simulink model "IEEE14_case"  (R2024b)
settings: Solver=FixedStepAuto  StartTime=0  StopTime=2  FixedStep=1e-7  RelTol=1e-3
values from neighbouring files (symbols this model uses):
  GFL_15_Bva = 0.009    [IEEE14_parameters.m]
  GFL_15_C_bus_pu = 7.179419    [IEEE14_parameters.m]
  GFL_15_f0 = 60    [IEEE14_parameters.m]
  GFL_15_I_id = 691.26967    [IEEE14_parameters.m]
  GFL_15_I_iq = 691.26967    [IEEE14_parameters.m]
  GFL_15_I_od = 45.2207    [IEEE14_parameters.m]
  GFL_15_I_oq = 45.2207    [IEEE14_parameters.m]
  GFL_15_I_pll = 0.78    [IEEE14_parameters.m]
  GFL_15_Kdi = 0.09    [IEEE14_parameters.m]
  GFL_15_Kdo = 0.9    [IEEE14_parameters.m]
  GFL_15_Kqi = 0.09    [IEEE14_parameters.m]
  GFL_15_Kqo = 0.9    [IEEE14_parameters.m]
  GFL_15_Lg_pu = 0.631447    [IEEE14_parameters.m]
  GFL_15_mode = 1    [IEEE14_parameters.m]
  GFL_15_P_id = 3.7166    [IEEE14_parameters.m]
  GFL_15_P_iq = 3.7166    [IEEE14_parameters.m]
  GFL_15_P_od = 0.4798    [IEEE14_parameters.m]
  GFL_15_P_oq = 0.4798    [IEEE14_parameters.m]
  GFL_15_P_pll = 290.42    [IEEE14_parameters.m]
  GFL_15_Qe_ref = 0.2    [IEEE14_parameters.m]
  GFL_15_Rg_pu = 0.024016    [IEEE14_parameters.m]
  GFL_15_Sbase = 1.000000e+4    (= 10000)    [IEEE14_parameters.m]
  GFL_15_Tdi = 0.01    [IEEE14_parameters.m]
  GFL_15_Tdo = 0.2    [IEEE14_parameters.m]
  GFL_15_Tqi = 0.01    [IEEE14_parameters.m]
  GFL_15_Tqo = 0.2    [IEEE14_parameters.m]
  GFL_15_Vbase = 380    [IEEE14_parameters.m]
  GFL_15_Vdc_ref = 1.011475    [IEEE14_parameters.m]
  GFL_15_Vdcbase = 700    [IEEE14_parameters.m]
  GFL_15_vq_ref = 0    [IEEE14_parameters.m]
  GFL_16_Bva = 0.002    [IEEE14_parameters.m]
  GFL_16_C_bus_pu = 7.179419    [IEEE14_parameters.m]
  GFL_16_f0 = 60    [IEEE14_parameters.m]
  GFL_16_I_id = 691.26967    [IEEE14_parameters.m]
  GFL_16_I_iq = 691.26967    [IEEE14_parameters.m]
  GFL_16_I_od = 45.2207    [IEEE14_parameters.m]
  GFL_16_I_oq = 45.2207    [IEEE14_parameters.m]
  GFL_16_I_pll = 0.78    [IEEE14_parameters.m]
  GFL_16_Kdi = 0.05    [IEEE14_parameters.m]
  GFL_16_Kdo = 0.5    [IEEE14_parameters.m]
  GFL_16_Kqi = 0.05    [IEEE14_parameters.m]
  GFL_16_Kqo = 0.5    [IEEE14_parameters.m]
  GFL_16_Lg_pu = 0.631447    [IEEE14_parameters.m]
  GFL_16_mode = 1    [IEEE14_parameters.m]
  GFL_16_P_id = 3.7166    [IEEE14_parameters.m]
  GFL_16_P_iq = 3.7166    [IEEE14_parameters.m]
  GFL_16_P_od = 0.4798    [IEEE14_parameters.m]
  GFL_16_P_oq = 0.4798    [IEEE14_parameters.m]
  GFL_16_P_pll = 290.42    [IEEE14_parameters.m]
  GFL_16_Qe_ref = 0.2    [IEEE14_parameters.m]
  GFL_16_Rg_pu = 0.024016    [IEEE14_parameters.m]
  GFL_16_Sbase = 1.000000e+4    (= 10000)    [IEEE14_parameters.m]
  GFL_16_Tdi = 0.01    [IEEE14_parameters.m]
  GFL_16_Tdo = 0.2    [IEEE14_parameters.m]
  GFL_16_Tqi = 0.01    [IEEE14_parameters.m]
  GFL_16_Tqo = 0.2    [IEEE14_parameters.m]
  GFL_16_Vbase = 380    [IEEE14_parameters.m]
  GFL_16_Vdc_ref = 1.01144    [IEEE14_parameters.m]
  GFL_16_Vdcbase = 700    [IEEE14_parameters.m]
  GFL_16_vq_ref = 0    [IEEE14_parameters.m]
  GFL_17_Bva = 0.002    [IEEE14_parameters.m]
  GFL_17_C_bus_pu = 7.179419    [IEEE14_parameters.m]
  GFL_17_f0 = 60    [IEEE14_parameters.m]
  GFL_17_I_id = 691.26967    [IEEE14_parameters.m]
  GFL_17_I_iq = 691.26967    [IEEE14_parameters.m]
  GFL_17_I_od = 45.2207    [IEEE14_parameters.m]
  GFL_17_I_oq = 45.2207    [IEEE14_parameters.m]
  GFL_17_I_pll = 0.78    [IEEE14_parameters.m]
  GFL_17_Kdi = 0.05    [IEEE14_parameters.m]
  GFL_17_Kdo = 0.5    [IEEE14_parameters.m]
  GFL_17_Kqi = 0.05    [IEEE14_parameters.m]
  GFL_17_Kqo = 0.5    [IEEE14_parameters.m]
  GFL_17_Lg_pu = 0.631447    [IEEE14_parameters.m]
  GFL_17_mode = 1    [IEEE14_parameters.m]
  GFL_17_P_id = 3.7166    [IEEE14_parameters.m]
  GFL_17_P_iq = 3.7166    [IEEE14_parameters.m]
  GFL_17_P_od = 0.4798    [IEEE14_parameters.m]
  GFL_17_P_oq = 0.4798    [IEEE14_parameters.m]
  GFL_17_P_pll = 290.42    [IEEE14_parameters.m]
  GFL_17_Qe_ref = 0.2    [IEEE14_parameters.m]
  GFL_17_Rg_pu = 0.024016    [IEEE14_parameters.m]
  GFL_17_Sbase = 1.000000e+4    (= 10000)    [IEEE14_parameters.m]
  GFL_17_Tdi = 0.01    [IEEE14_parameters.m]
  GFL_17_Tdo = 0.2    [IEEE14_parameters.m]
  GFL_17_Tqi = 0.01    [IEEE14_parameters.m]
  GFL_17_Tqo = 0.2    [IEEE14_parameters.m]
  GFL_17_Vbase = 380    [IEEE14_parameters.m]
  GFL_17_Vdc_ref = 1.011632    [IEEE14_parameters.m]
  GFL_17_Vdcbase = 700    [IEEE14_parameters.m]
  GFL_17_vq_ref = 0    [IEEE14_parameters.m]
  GFL_18_Bva = 0.002    [IEEE14_parameters.m]
  GFL_18_C_bus_pu = 7.179419    [IEEE14_parameters.m]
  GFL_18_f0 = 60    [IEEE14_parameters.m]
  GFL_18_I_id = 691.26967    [IEEE14_parameters.m]
  GFL_18_I_iq = 691.26967    [IEEE14_parameters.m]
  GFL_18_I_od = 45.2207    [IEEE14_parameters.m]
  GFL_18_I_oq = 45.2207    [IEEE14_parameters.m]
  GFL_18_I_pll = 0.78    [IEEE14_parameters.m]
  GFL_18_Kdi = 0.05    [IEEE14_parameters.m]
  GFL_18_Kdo = 0.5    [IEEE14_parameters.m]
  GFL_18_Kqi = 0.05    [IEEE14_parameters.m]
  GFL_18_Kqo = 0.5    [IEEE14_parameters.m]
  GFL_18_Lg_pu = 0.631447    [IEEE14_parameters.m]
  GFL_18_mode = 1    [IEEE14_parameters.m]
  GFL_18_P_id = 3.7166    [IEEE14_parameters.m]
  GFL_18_P_iq = 3.7166    [IEEE14_parameters.m]
  GFL_18_P_od = 0.4798    [IEEE14_parameters.m]
  GFL_18_P_oq = 0.4798    [IEEE14_parameters.m]
  GFL_18_P_pll = 290.42    [IEEE14_parameters.m]
  GFL_18_Qe_ref = 0.2    [IEEE14_parameters.m]
  GFL_18_Rg_pu = 0.024016    [IEEE14_parameters.m]
  GFL_18_Sbase = 1.000000e+4    (= 10000)    [IEEE14_parameters.m]
  GFL_18_Tdi = 0.01    [IEEE14_parameters.m]
  GFL_18_Tdo = 0.2    [IEEE14_parameters.m]
  GFL_18_Tqi = 0.01    [IEEE14_parameters.m]
  GFL_18_Tqo = 0.2    [IEEE14_parameters.m]
  GFL_18_Vbase = 380    [IEEE14_parameters.m]
  GFL_18_Vdc_ref = 1.011572    [IEEE14_parameters.m]
  GFL_18_Vdcbase = 700    [IEEE14_parameters.m]
  GFL_18_vq_ref = 0    [IEEE14_parameters.m]
  ... (+180 more)
(part 6 of 25)

== system IEEE14_case/AC_1/d_id_line_7_9_block ==
  note: d_id_line_7_9 in case14gfl
      | $376.991118430775\,\mathrm{iq}_{\mathrm{line},7,9}+3426.88045114785\,\mathrm{vd}_{\mathrm{bus},7}-3426.88045114785\,\mathrm{vd}_{\mathrm{bus},9}$
      | Automatically generated on 2025-10-09 21:39:39 .
  State_iq_line_7_9_66432 : Inport
  State_vd_bus_7_8bd9d : Inport  Port=2
  State_vd_bus_9_0bd7a : Inport  Port=3
  Add_05699 : Sum
  Constant_3426.88045114785_50b4f : Constant  Value=3426.88045114785
  Constant_3426.88045114785_9598e : Constant  Value=3426.88045114785
  Constant_376.991118430775_0858e : Constant  Value=376.991118430775
  Product_57b21 : Product
  Product_92e7d : Product
  Product_acf4f : Product
  Subtract_c4abe : Sum  Inputs=+-
  Blockout_d_id_line_7_9_bf772 : Outport
  wires:
  State_iq_line_7_9_66432/1 -> Product_57b21/2
  Constant_376.991118430775_0858e/1 -> Product_57b21/1
  Constant_3426.88045114785_50b4f/1 -> Product_92e7d/1
  Product_92e7d/1 -> Add_05699/2
  State_vd_bus_7_8bd9d/1 -> Product_92e7d/2
  Product_57b21/1 -> Add_05699/1
  Product_acf4f/1 -> Subtract_c4abe/2
  Constant_3426.88045114785_9598e/1 -> Product_acf4f/1
  State_vd_bus_9_0bd7a/1 -> Product_acf4f/2
  Add_05699/1 -> Subtract_c4abe/1
  Subtract_c4abe/1 -> Blockout_d_id_line_7_9_bf772/1

== system IEEE14_case/AC_1/d_id_line_9_10_block ==
  note: d_id_line_9_10 in case14gfl
      | $376.991118430775\,\mathrm{iq}_{\mathrm{line},9,10}-141.918194997431\,\mathrm{id}_{\mathrm{line},9,10}+4461.43335421036\,\mathrm{vd}_{\mathrm{bus},9}-4461.43335421036\,\mathrm{vd}_{\mathrm{bus},10}$
      | Automatically generated on 2025-10-09 21:39:41 .
  State_id_line_9_10_959cd : Inport
  State_iq_line_9_10_22e13 : Inport  Port=2
  State_vd_bus_10_33748 : Inport  Port=3
  State_vd_bus_9_919cb : Inport  Port=4
  Add_7717b : Sum
  Add_e4eab : Sum
  Constant_-141.918194997431_d6c81 : Constant  Value=-141.918194997431
  Constant_376.991118430775_9f4c1 : Constant  Value=376.991118430775
  Constant_4461.43335421036_3f7bf : Constant  Value=4461.43335421036
  Constant_4461.43335421036_5c0f1 : Constant  Value=4461.43335421036
  Product_24143 : Product
  Product_2f834 : Product
  Product_723bb : Product
  Product_a30df : Product
  Subtract_8e61d : Sum  Inputs=+-
  Blockout_d_id_line_9_10_ec156 : Outport
  wires:
  Constant_-141.918194997431_d6c81/1 -> Product_a30df/1
  Product_a30df/1 -> Add_7717b/1
  State_id_line_9_10_959cd/1 -> Product_a30df/2
  Constant_376.991118430775_9f4c1/1 -> Product_24143/1
  Product_24143/1 -> Add_7717b/2
  Product_723bb/1 -> Subtract_8e61d/2
  Constant_4461.43335421036_3f7bf/1 -> Product_723bb/1
  State_iq_line_9_10_22e13/1 -> Product_24143/2
  State_vd_bus_10_33748/1 -> Product_723bb/2
  Add_7717b/1 -> Subtract_8e61d/1
  Constant_4461.43335421036_5c0f1/1 -> Product_2f834/1
  State_vd_bus_9_919cb/1 -> Product_2f834/2
  Subtract_8e61d/1 -> Add_e4eab/1
  Product_2f834/1 -> Add_e4eab/2
  Add_e4eab/1 -> Blockout_d_id_line_9_10_ec156/1

== system IEEE14_case/AC_1/d_id_line_9_14_block ==
  note: d_id_line_9_14 in case14gfl
      | $376.991118430775\,\mathrm{iq}_{\mathrm{line},9,14}-177.229606715496\,\mathrm{id}_{\mathrm{line},9,14}+1394.30105196677\,\mathrm{vd}_{\mathrm{bus},9}-1394.30105196677\,\mathrm{vd}_{\mathrm{bus},14}$
      | Automatically generated on 2025-10-09 21:39:44 .
  State_id_line_9_14_b515e : Inport
  State_iq_line_9_14_72453 : Inport  Port=2
  State_vd_bus_14_60cbb : Inport  Port=3
  State_vd_bus_9_8eb23 : Inport  Port=4
  Add_65adc : Sum
  Add_8bfe2 : Sum
  Constant_-177.229606715496_fa7d8 : Constant  Value=-177.229606715496
  Constant_1394.30105196677_66f77 : Constant  Value=1394.30105196677
  Constant_1394.30105196677_7cf1b : Constant  Value=1394.30105196677
  Constant_376.991118430775_d6f44 : Constant  Value=376.991118430775
  Product_28f27 : Product
  Product_78e64 : Product
  Product_8a520 : Product
  Product_c0cd1 : Product
  Subtract_feb9f : Sum  Inputs=+-
  Blockout_d_id_line_9_14_6ccdc : Outport
  wires:
  Constant_-177.229606715496_fa7d8/1 -> Product_c0cd1/1
  Product_c0cd1/1 -> Add_8bfe2/1
  State_id_line_9_14_b515e/1 -> Product_c0cd1/2
  Constant_376.991118430775_d6f44/1 -> Product_78e64/1
  State_iq_line_9_14_72453/1 -> Product_78e64/2
  Product_78e64/1 -> Add_8bfe2/2
  State_vd_bus_14_60cbb/1 -> Product_8a520/2
  Product_8a520/1 -> Subtract_feb9f/2
  Constant_1394.30105196677_66f77/1 -> Product_8a520/1
  Add_8bfe2/1 -> Subtract_feb9f/1
  Product_28f27/1 -> Add_65adc/2
  Constant_1394.30105196677_7cf1b/1 -> Product_28f27/1
  State_vd_bus_9_8eb23/1 -> Product_28f27/2
  Subtract_feb9f/1 -> Add_65adc/1
  Add_65adc/1 -> Blockout_d_id_line_9_14_6ccdc/1

== system IEEE14_case/AC_1/d_id_load_10_block ==
  note: d_id_load_10 in case14gfl
      | $376.991118430775\,\mathrm{iq}_{\mathrm{load},10}-584.986218254651\,\mathrm{id}_{\mathrm{load},10}+60.6278129379132\,\mathrm{vd}_{\mathrm{bus},10}$
      | Automatically generated on 2025-10-09 21:39:01 .
  State_id_load_10_31e9c : Inport
  State_iq_load_10_87559 : Inport  Port=2
  State_vd_bus_10_d1446 : Inport  Port=3
  Add_12c63 : Sum
  Add_264d0 : Sum
  Constant_-584.986218254651_122b3 : Constant  Value=-584.986218254651
  Constant_376.991118430775_eb9de : Constant  Value=376.991118430775
  Constant_60.6278129379132_b56b3 : Constant  Value=60.6278129379132
  Product_20162 : Product
  Product_6cc79 : Product
  Product_c214a : Product
  Blockout_d_id_load_10_a8029 : Outport
  wires:
  Constant_-584.986218254651_122b3/1 -> Product_6cc79/1
  Constant_376.991118430775_eb9de/1 -> Product_c214a/1
  Product_c214a/1 -> Add_264d0/2
  Product_6cc79/1 -> Add_264d0/1
  State_id_load_10_31e9c/1 -> Product_6cc79/2
  Product_20162/1 -> Add_12c63/2
  Constant_60.6278129379132_b56b3/1 -> Product_20162/1
  State_iq_load_10_87559/1 -> Product_c214a/2
  State_vd_bus_10_d1446/1 -> Product_20162/2
  Add_264d0/1 -> Add_12c63/1
  Add_12c63/1 -> Blockout_d_id_load_10_a8029/1

== system IEEE14_case/AC_1/d_id_load_11_block ==
  note: d_id_load_11 in case14gfl
      | $376.991118430775\,\mathrm{iq}_{\mathrm{load},11}-733.038285837618\,\mathrm{id}_{\mathrm{load},11}+26.9582940185634\,\mathrm{vd}_{\mathrm{bus},11}$
      | Automatically generated on 2025-10-09 21:39:03 .
  State_id_load_11_628b0 : Inport
  State_iq_load_11_d9a12 : Inport  Port=2
  State_vd_bus_11_633a4 : Inport  Port=3
  Add_a764a : Sum
  Add_f90df : Sum
  Constant_-733.038285837618_2787a : Constant  Value=-733.038285837618
  Constant_26.9582940185634_112f4 : Constant  Value=26.9582940185634
  Constant_376.991118430775_74a6d : Constant  Value=376.991118430775
  Product_38bd8 : Product
  Product_9e0fa : Product
  Product_cb022 : Product
  Blockout_d_id_load_11_86202 : Outport
  wires:
  Constant_-733.038285837618_2787a/1 -> Product_9e0fa/1
  Product_9e0fa/1 -> Add_a764a/1
  State_id_load_11_628b0/1 -> Product_9e0fa/2
  Constant_376.991118430775_74a6d/1 -> Product_38bd8/1
  Product_38bd8/1 -> Add_a764a/2
  State_iq_load_11_d9a12/1 -> Product_38bd8/2
  Product_cb022/1 -> Add_f90df/2
  Constant_26.9582940185634_112f4/1 -> Product_cb022/1
  State_vd_bus_11_633a4/1 -> Product_cb022/2
  Add_a764a/1 -> Add_f90df/1
  Add_f90df/1 -> Blockout_d_id_load_11_86202/1

== system IEEE14_case/AC_1/d_id_load_12_block ==
  note: d_id_load_12 in case14gfl
      | $376.991118430775\,\mathrm{iq}_{\mathrm{load},12}-1437.27863901733\,\mathrm{id}_{\mathrm{load},12}+77.623450441014\,\mathrm{vd}_{\mathrm{bus},12}$
      | Automatically generated on 2025-10-09 21:39:05 .
  State_id_load_12_be97f : Inport
  State_iq_load_12_84390 : Inport  Port=2
  State_vd_bus_12_f1be8 : Inport  Port=3
  Add_ea2c6 : Sum
  Add_f3c7f : Sum
  Constant_-1437.27863901733_a3140 : Constant  Value=-1437.27863901733
  Constant_376.991118430775_ad15b : Constant  Value=376.991118430775
  Constant_77.623450441014_c24b0 : Constant  Value=77.623450441014
  Product_9bb77 : Product
  Product_e53cc : Product
  Product_eef8b : Product
  Blockout_d_id_load_12_58f44 : Outport
  wires:
  Constant_-1437.27863901733_a3140/1 -> Product_eef8b/1
  Constant_376.991118430775_ad15b/1 -> Product_e53cc/1
  Product_e53cc/1 -> Add_f3c7f/2
  Product_eef8b/1 -> Add_f3c7f/1
  State_id_load_12_be97f/1 -> Product_eef8b/2
  Product_9bb77/1 -> Add_ea2c6/2
  Constant_77.623450441014_c24b0/1 -> Product_9bb77/1
  State_iq_load_12_84390/1 -> Product_e53cc/2
  State_vd_bus_12_f1be8/1 -> Product_9bb77/2
  Add_f3c7f/1 -> Add_ea2c6/1
  Add_ea2c6/1 -> Blockout_d_id_load_12_58f44/1

== system IEEE14_case/AC_1/d_id_load_13_block ==
  note: d_id_load_13 in case14gfl
      | $376.991118430775\,\mathrm{iq}_{\mathrm{load},13}-877.479327381977\,\mathrm{id}_{\mathrm{load},13}+118.242352238424\,\mathrm{vd}_{\mathrm{bus},13}$
      | Automatically generated on 2025-10-09 21:39:07 .
  State_id_load_13_999eb : Inport
  State_iq_load_13_edcc2 : Inport  Port=2
  State_vd_bus_13_31285 : Inport  Port=3
  Add_51588 : Sum
  Add_631ba : Sum
  Constant_-877.479327381977_345b2 : Constant  Value=-877.479327381977
  Constant_118.242352238424_9562b : Constant  Value=118.242352238424
  Constant_376.991118430775_9a86e : Constant  Value=376.991118430775
  Product_052eb : Product
  Product_74f7d : Product
  Product_e65fd : Product
  Blockout_d_id_load_13_e8012 : Outport
  wires:
  Constant_-877.479327381977_345b2/1 -> Product_e65fd/1
  Product_e65fd/1 -> Add_631ba/1
  State_id_load_13_999eb/1 -> Product_e65fd/2
  Constant_376.991118430775_9a86e/1 -> Product_052eb/1
  Product_052eb/1 -> Add_631ba/2
  State_iq_load_13_edcc2/1 -> Product_052eb/2
  Product_74f7d/1 -> Add_51588/2
  Constant_118.242352238424_9562b/1 -> Product_74f7d/1
  State_vd_bus_13_31285/1 -> Product_74f7d/2
  Add_631ba/1 -> Add_51588/1
  Add_51588/1 -> Blockout_d_id_load_13_e8012/1

== system IEEE14_case/AC_1/d_id_load_14_block ==
  note: d_id_load_14 in case14gfl
      | $376.991118430775\,\mathrm{iq}_{\mathrm{load},14}-1123.43353292371\,\mathrm{id}_{\mathrm{load},14}+156.099712947555\,\mathrm{vd}_{\mathrm{bus},14}$
      | Automatically generated on 2025-10-09 21:39:09 .
  State_id_load_14_2e0ae : Inport
  State_iq_load_14_2d6b8 : Inport  Port=2
  State_vd_bus_14_a8c17 : Inport  Port=3
  Add_0dee3 : Sum
  Add_46003 : Sum
  Constant_-1123.43353292371_3948e : Constant  Value=-1123.43353292371
  Constant_156.099712947555_0eca3 : Constant  Value=156.099712947555
  Constant_376.991118430775_f46ef : Constant  Value=376.991118430775
  Product_0c414 : Product
  Product_7a545 : Product
  Product_d9ff2 : Product
  Blockout_d_id_load_14_efc39 : Outport
  wires:
  Constant_-1123.43353292371_3948e/1 -> Product_d9ff2/1
  Constant_376.991118430775_f46ef/1 -> Product_0c414/1
  Product_0c414/1 -> Add_46003/2
  Product_d9ff2/1 -> Add_46003/1
  State_id_load_14_2e0ae/1 -> Product_d9ff2/2
  Product_7a545/1 -> Add_0dee3/2
  Constant_156.099712947555_0eca3/1 -> Product_7a545/1
  State_iq_load_14_2d6b8/1 -> Product_0c414/2
  State_vd_bus_14_a8c17/1 -> Product_7a545/2
  Add_46003/1 -> Add_0dee3/1
  Add_0dee3/1 -> Blockout_d_id_load_14_efc39/1

== system IEEE14_case/AC_1/d_id_load_2_block ==
  note: d_id_load_2 in case14gfl
      | $376.991118430775\,\mathrm{iq}_{\mathrm{load},2}-644.150178736049\,\mathrm{id}_{\mathrm{load},2}+171.84447318187\,\mathrm{vd}_{\mathrm{bus},2}$
      | Automatically generated on 2025-10-09 21:38:50 .
  State_id_load_2_f170a : Inport
  State_iq_load_2_a0763 : Inport  Port=2
  State_vd_bus_2_22b83 : Inport  Port=3
  Add_ac749 : Sum
  Add_f656d : Sum
  Constant_-644.150178736049_cb8ea : Constant  Value=-644.150178736049
  Constant_171.84447318187_2f5b1 : Constant  Value=171.84447318187
  Constant_376.991118430775_e780b : Constant  Value=376.991118430775
  Product_2b33f : Product
  Product_51d22 : Product
  Product_71ca9 : Product
  Blockout_d_id_load_2_a876e : Outport
  wires:
  State_vd_bus_2_22b83/1 -> Product_2b33f/2
  Constant_-644.150178736049_cb8ea/1 -> Product_71ca9/1
  Product_71ca9/1 -> Add_f656d/1
  Product_2b33f/1 -> Add_ac749/2
  Constant_171.84447318187_2f5b1/1 -> Product_2b33f/1
  State_id_load_2_f170a/1 -> Product_71ca9/2
  Constant_376.991118430775_e780b/1 -> Product_51d22/1
  Product_51d22/1 -> Add_f656d/2
  State_iq_load_2_a0763/1 -> Product_51d22/2
  Add_f656d/1 -> Add_ac749/1
  Add_ac749/1 -> Blockout_d_id_load_2_a876e/1

== system IEEE14_case/AC_1/d_id_load_3_block ==
  note: d_id_load_3 in case14gfl
      | $376.991118430775\,\mathrm{iq}_{\mathrm{load},3}-1869.08228190416\,\mathrm{id}_{\mathrm{load},3}+1796.20019807427\,\mathrm{vd}_{\mathrm{bus},3}$
      | Automatically generated on 2025-10-09 21:38:52 .
  State_id_load_3_166da : Inport
  State_iq_load_3_14c81 : Inport  Port=2
  State_vd_bus_3_b5bb0 : Inport  Port=3
  Add_11df1 : Sum
  Add_2f39e : Sum
  Constant_-1869.08228190416_77d20 : Constant  Value=-1869.08228190416
  Constant_1796.20019807427_560b3 : Constant  Value=1796.20019807427
  Constant_376.991118430775_53ed6 : Constant  Value=376.991118430775
  Product_24e08 : Product
  Product_292dd : Product
  Product_56913 : Product
  Blockout_d_id_load_3_c7879 : Outport
  wires:
  Constant_-1869.08228190416_77d20/1 -> Product_56913/1
  Constant_376.991118430775_53ed6/1 -> Product_292dd/1
  Product_292dd/1 -> Add_11df1/2
  Product_56913/1 -> Add_11df1/1
  State_id_load_3_166da/1 -> Product_56913/2
  State_iq_load_3_14c81/1 -> Product_292dd/2
  Product_24e08/1 -> Add_2f39e/2
  Constant_1796.20019807427_560b3/1 -> Product_24e08/1
  State_vd_bus_3_b5bb0/1 -> Product_24e08/2
  Add_11df1/1 -> Add_2f39e/1
  Add_2f39e/1 -> Blockout_d_id_load_3_c7879/1

== system IEEE14_case/AC_1/d_id_load_4_block ==
  note: d_id_load_4 in case14gfl
      | $376.991118430775\,\mathrm{iq}_{\mathrm{load},4}-4620.55781051053\,\mathrm{id}_{\mathrm{load},4}+2007.66181460144\,\mathrm{vd}_{\mathrm{bus},4}$
      | Automatically generated on 2025-10-09 21:38:53 .
  State_id_load_4_9125b : Inport
  State_iq_load_4_3a649 : Inport  Port=2
  State_vd_bus_4_11e1c : Inport  Port=3
  Add_98740 : Sum
  Add_fad10 : Sum
  Constant_-4620.55781051053_1570f : Constant  Value=-4620.55781051053
  Constant_2007.66181460144_8008a : Constant  Value=2007.66181460144
  Constant_376.991118430775_a3c5a : Constant  Value=376.991118430775
  Product_4410f : Product
  Product_533ea : Product
  Product_69609 : Product
  Blockout_d_id_load_4_eca8f : Outport
  wires:
  Constant_-4620.55781051053_1570f/1 -> Product_4410f/1
  Product_4410f/1 -> Add_fad10/1
  State_id_load_4_9125b/1 -> Product_4410f/2
  Constant_376.991118430775_a3c5a/1 -> Product_533ea/1
  Product_533ea/1 -> Add_fad10/2
  State_iq_load_4_3a649/1 -> Product_533ea/2
  Product_69609/1 -> Add_98740/2
  Constant_2007.66181460144_8008a/1 -> Product_69609/1
  State_vd_bus_4_11e1c/1 -> Product_69609/2
  Add_fad10/1 -> Add_98740/1
  Add_98740/1 -> Blockout_d_id_load_4_eca8f/1

== system IEEE14_case/AC_1/d_id_load_5_block ==
  note: d_id_load_5 in case14gfl
      | $376.991118430775\,\mathrm{iq}_{\mathrm{load},5}-1790.70781254618\,\mathrm{id}_{\mathrm{load},5}+126.842875202809\,\mathrm{vd}_{\mathrm{bus},5}$
      | Automatically generated on 2025-10-09 21:38:55 .
  State_id_load_5_82a6e : Inport
  State_iq_load_5_f0bf8 : Inport  Port=2
  State_vd_bus_5_96189 : Inport  Port=3
  Add_a3ea9 : Sum
  Add_b8d13 : Sum
  Constant_-1790.70781254618_4bfc6 : Constant  Value=-1790.70781254618
  Constant_126.842875202809_6dbf9 : Constant  Value=126.842875202809
  Constant_376.991118430775_2243d : Constant  Value=376.991118430775
  Product_2d359 : Product
  Product_c73da : Product
  Product_e913f : Product
  Blockout_d_id_load_5_99e2f : Outport
  wires:
  Constant_-1790.70781254618_4bfc6/1 -> Product_2d359/1
  Product_2d359/1 -> Add_a3ea9/1
  State_id_load_5_82a6e/1 -> Product_2d359/2
  Constant_376.991118430775_2243d/1 -> Product_e913f/1
  Product_e913f/1 -> Add_a3ea9/2
  Product_c73da/1 -> Add_b8d13/2
  Constant_126.842875202809_6dbf9/1 -> Product_c73da/1
  State_iq_load_5_f0bf8/1 -> Product_e913f/2
  State_vd_bus_5_96189/1 -> Product_c73da/2
  Add_a3ea9/1 -> Add_b8d13/1
  Add_b8d13/1 -> Blockout_d_id_load_5_99e2f/1

== system IEEE14_case/AC_1/d_id_load_6_block ==
  note: d_id_load_6 in case14gfl
      | $376.991118430775\,\mathrm{iq}_{\mathrm{load},6}-562.973403523291\,\mathrm{id}_{\mathrm{load},6}+79.7688488749381\,\mathrm{vd}_{\mathrm{bus},6}$
      | Automatically generated on 2025-10-09 21:38:57 .
  State_id_load_6_6a8f0 : Inport
  State_iq_load_6_5ea6c : Inport  Port=2
  State_vd_bus_6_858b4 : Inport  Port=3
  Add_4515b : Sum
  Add_bdd66 : Sum
  Constant_-562.973403523291_a98db : Constant  Value=-562.973403523291
  Constant_376.991118430775_cf668 : Constant  Value=376.991118430775
  Constant_79.7688488749381_83b4c : Constant  Value=79.7688488749381
  Product_32683 : Product
  Product_56242 : Product
  Product_af3d3 : Product
  Blockout_d_id_load_6_d0eb4 : Outport
  wires:
  State_vd_bus_6_858b4/1 -> Product_af3d3/2
  Constant_-562.973403523291_a98db/1 -> Product_56242/1
  Product_af3d3/1 -> Add_4515b/2
  Constant_79.7688488749381_83b4c/1 -> Product_af3d3/1
  Product_56242/1 -> Add_bdd66/1
  State_id_load_6_6a8f0/1 -> Product_56242/2
  Constant_376.991118430775_cf668/1 -> Product_32683/1
  Product_32683/1 -> Add_bdd66/2
  State_iq_load_6_5ea6c/1 -> Product_32683/2
  Add_bdd66/1 -> Add_4515b/1
  Add_4515b/1 -> Blockout_d_id_load_6_d0eb4/1

== system IEEE14_case/AC_1/d_id_load_9_block ==
  note: d_id_load_9 in case14gfl
      | $376.991118430775\,\mathrm{iq}_{\mathrm{load},9}-669.954096006498\,\mathrm{id}_{\mathrm{load},9}+214.658794552347\,\mathrm{vd}_{\mathrm{bus},9}$
      | Automatically generated on 2025-10-09 21:38:59 .
  State_id_load_9_8af8e : Inport
  State_iq_load_9_3ccc7 : Inport  Port=2
  State_vd_bus_9_e4c71 : Inport  Port=3
  Add_3940c : Sum
  Add_4ba24 : Sum
  Constant_-669.954096006498_3b62a : Constant  Value=-669.954096006498
  Constant_214.658794552347_fc8fa : Constant  Value=214.658794552347
  Constant_376.991118430775_314db : Constant  Value=376.991118430775
  Product_17e7f : Product
  Product_5a290 : Product
  Product_7714d : Product
  Blockout_d_id_load_9_e6f54 : Outport
  wires:
  Constant_-669.954096006498_3b62a/1 -> Product_17e7f/1
  Constant_376.991118430775_314db/1 -> Product_7714d/1
  Product_7714d/1 -> Add_4ba24/2
  Product_17e7f/1 -> Add_4ba24/1
  State_id_load_9_8af8e/1 -> Product_17e7f/2
  State_iq_load_9_3ccc7/1 -> Product_7714d/2
  Product_5a290/1 -> Add_3940c/2
  Constant_214.658794552347_fc8fa/1 -> Product_5a290/1
  State_vd_bus_9_e4c71/1 -> Product_5a290/2
  Add_4ba24/1 -> Add_3940c/1
  Add_3940c/1 -> Blockout_d_id_load_9_e6f54/1

== system IEEE14_case/AC_1/d_iq_line_10_11_block ==
  note: d_iq_line_10_11 in case14gfl
      | $1962.77981168728\,\mathrm{vq}_{\mathrm{bus},10}-161.046083548941\,\mathrm{iq}_{\mathrm{line},10,11}-376.991118430775\,\mathrm{id}_{\mathrm{line},10,11}-1962.77981168728\,\mathrm{vq}_{\mathrm{bus},11}$
      | Automatically generated on 2025-10-09 21:39:47 .
  State_id_line_10_11_672ad : Inport
  State_iq_line_10_11_0ead8 : Inport  Port=2
  State_vq_bus_10_f1a56 : Inport  Port=3
  State_vq_bus_11_9096b : Inport  Port=4
  Add_6aecc : Sum
  Constant_-376.991118430775_b34af : Constant  Value=-376.991118430775
  Constant_161.046083548941_50a44 : Constant  Value=161.046083548941
  Constant_1962.77981168728_af3f4 : Constant  Value=1962.77981168728
  Constant_1962.77981168728_c1513 : Constant  Value=1962.77981168728
  Product_41ecc : Product
  Product_603aa : Product
  Product_8f18b : Product
  Product_d0233 : Product
  Subtract_0b8df : Sum  Inputs=+-
  Subtract_a156b : Sum  Inputs=+-
  Blockout_d_iq_line_10_11_8dcae : Outport
  wires:
  State_vq_bus_10_f1a56/1 -> Product_603aa/2
  Constant_-376.991118430775_b34af/1 -> Product_8f18b/1
  Product_603aa/1 -> Add_6aecc/2
  Constant_1962.77981168728_c1513/1 -> Product_603aa/1
  Product_8f18b/1 -> Subtract_a156b/1
  State_id_line_10_11_672ad/1 -> Product_8f18b/2
  Constant_161.046083548941_50a44/1 -> Product_41ecc/1
  Product_41ecc/1 -> Subtract_a156b/2
  State_iq_line_10_11_0ead8/1 -> Product_41ecc/2
  Subtract_a156b/1 -> Add_6aecc/1
  Constant_1962.77981168728_af3f4/1 -> Product_d0233/1
  State_vq_bus_11_9096b/1 -> Product_d0233/2
  Add_6aecc/1 -> Subtract_0b8df/1
  Product_d0233/1 -> Subtract_0b8df/2
  Subtract_0b8df/1 -> Blockout_d_iq_line_10_11_8dcae/1

== system IEEE14_case/AC_1/d_iq_line_11_15_block ==
  note: d_iq_line_11_15 in case14gfl
      | $538.558740615393\,\mathrm{vq}_{\mathrm{bus},11}-32.3135244369236\,\mathrm{iq}_{\mathrm{line},11,15}-376.991118430775\,\mathrm{id}_{\mathrm{line},11,15}-538.558740615393\,\mathrm{vq}_{\mathrm{bus},15}$
      | Automatically generated on 2025-10-09 21:39:54 .
  State_id_line_11_15_35576 : Inport
  State_iq_line_11_15_b5696 : Inport  Port=2
  State_vq_bus_11_fe1e1 : Inport  Port=3
  State_vq_bus_15_132fc : Inport  Port=4
  Add_80d1b : Sum
  Constant_-376.991118430775_7b4f0 : Constant  Value=-376.991118430775
  Constant_32.3135244369236_189ae : Constant  Value=32.3135244369236
  Constant_538.558740615393_0a8c4 : Constant  Value=538.558740615393
  Constant_538.558740615393_61c3b : Constant  Value=538.558740615393
  Product_05ae1 : Product
  Product_4ef2d : Product
  Product_7decd : Product
  Product_9f0dc : Product
  Subtract_e9dd0 : Sum  Inputs=+-
  Subtract_ec636 : Sum  Inputs=+-
  Blockout_d_iq_line_11_15_665a1 : Outport
  wires:
  Constant_-376.991118430775_7b4f0/1 -> Product_05ae1/1
  Constant_32.3135244369236_189ae/1 -> Product_9f0dc/1
  Product_9f0dc/1 -> Subtract_ec636/2
  State_id_line_11_15_35576/1 -> Product_05ae1/2
  Product_4ef2d/1 -> Add_80d1b/2
  Constant_538.558740615393_61c3b/1 -> Product_4ef2d/1
  State_iq_line_11_15_b5696/1 -> Product_9f0dc/2
  Product_05ae1/1 -> Subtract_ec636/1
  State_vq_bus_11_fe1e1/1 -> Product_4ef2d/2
  Subtract_ec636/1 -> Add_80d1b/1
  Product_7decd/1 -> Subtract_e9dd0/2
  Constant_538.558740615393_0a8c4/1 -> Product_7decd/1
  Add_80d1b/1 -> Subtract_e9dd0/1
  State_vq_bus_15_132fc/1 -> Product_7decd/2
  Subtract_e9dd0/1 -> Blockout_d_iq_line_11_15_665a1/1

== system IEEE14_case/AC_1/d_iq_line_12_13_block ==
  note: d_iq_line_12_13 in case14gfl
      | $1886.08724450058\,\mathrm{vq}_{\mathrm{bus},12}-416.674394055067\,\mathrm{iq}_{\mathrm{line},12,13}-376.991118430775\,\mathrm{id}_{\mathrm{line},12,13}-1886.08724450058\,\mathrm{vq}_{\mathrm{bus},13}$
      | Automatically generated on 2025-10-09 21:39:49 .
  State_id_line_12_13_b8b65 : Inport
  State_iq_line_12_13_eef70 : Inport  Port=2
  State_vq_bus_12_5dc3a : Inport  Port=3
  State_vq_bus_13_52e4e : Inport  Port=4
  Add_2db85 : Sum
  Constant_-376.991118430775_c97bc : Constant  Value=-376.991118430775
  Constant_1886.08724450058_baded : Constant  Value=1886.08724450058
  Constant_1886.08724450058_d9ce0 : Constant  Value=1886.08724450058
  Constant_416.674394055067_0198a : Constant  Value=416.674394055067
  Product_6ef9c : Product
  Product_c265c : Product
  Product_f0655 : Product
  Product_f9b6b : Product
  Subtract_9096b : Sum  Inputs=+-
  Subtract_fbe27 : Sum  Inputs=+-
  Blockout_d_iq_line_12_13_64197 : Outport
  wires:
  State_id_line_12_13_b8b65/1 -> Product_c265c/2
  Constant_-376.991118430775_c97bc/1 -> Product_c265c/1
  Constant_416.674394055067_0198a/1 -> Product_f0655/1
  State_iq_line_12_13_eef70/1 -> Product_f0655/2
  Product_f0655/1 -> Subtract_fbe27/2
  Product_c265c/1 -> Subtract_fbe27/1
  Product_6ef9c/1 -> Add_2db85/2
  Constant_1886.08724450058_d9ce0/1 -> Product_6ef9c/1
  State_vq_bus_12_5dc3a/1 -> Product_6ef9c/2
  Subtract_fbe27/1 -> Add_2db85/1
  Product_f9b6b/1 -> Subtract_9096b/2
  Constant_1886.08724450058_baded/1 -> Product_f9b6b/1
  State_vq_bus_13_52e4e/1 -> Product_f9b6b/2
  Add_2db85/1 -> Subtract_9096b/1
  Subtract_9096b/1 -> Blockout_d_iq_line_12_13_64197/1

== system IEEE14_case/AC_1/d_iq_line_12_16_block ==
  note: d_iq_line_12_16 in case14gfl
      | $538.558740615393\,\mathrm{vq}_{\mathrm{bus},12}-32.3135244369236\,\mathrm{iq}_{\mathrm{line},12,16}-376.991118430775\,\mathrm{id}_{\mathrm{line},12,16}-538.558740615393\,\mathrm{vq}_{\mathrm{bus},16}$
      | Automatically generated on 2025-10-09 21:39:56 .
  State_id_line_12_16_8add4 : Inport
  State_iq_line_12_16_8bc6b : Inport  Port=2
  State_vq_bus_12_58935 : Inport  Port=3
  State_vq_bus_16_f8d4f : Inport  Port=4
  Add_622af : Sum
  Constant_-376.991118430775_20b77 : Constant  Value=-376.991118430775
  Constant_32.3135244369236_b5758 : Constant  Value=32.3135244369236
  Constant_538.558740615393_10bd8 : Constant  Value=538.558740615393
  Constant_538.558740615393_439c2 : Constant  Value=538.558740615393
  Product_23ba4 : Product
  Product_2c296 : Product
  Product_4adc3 : Product
  Product_85c6d : Product
  Subtract_84366 : Sum  Inputs=+-
  Subtract_86653 : Sum  Inputs=+-
  Blockout_d_iq_line_12_16_95ad9 : Outport
  wires:
  Constant_-376.991118430775_20b77/1 -> Product_23ba4/1
  Product_23ba4/1 -> Subtract_86653/1
  State_id_line_12_16_8add4/1 -> Product_23ba4/2
  Constant_32.3135244369236_b5758/1 -> Product_4adc3/1
  Product_4adc3/1 -> Subtract_86653/2
  State_iq_line_12_16_8bc6b/1 -> Product_4adc3/2
  Subtract_84366/1 -> Blockout_d_iq_line_12_16_95ad9/1
  Product_2c296/1 -> Add_622af/2
  Constant_538.558740615393_439c2/1 -> Product_2c296/1
  State_vq_bus_12_58935/1 -> Product_2c296/2
  Subtract_86653/1 -> Add_622af/1
  Constant_538.558740615393_10bd8/1 -> Product_85c6d/1
  State_vq_bus_16_f8d4f/1 -> Product_85c6d/2
  Add_622af/1 -> Subtract_84366/1
  Product_85c6d/1 -> Subtract_84366/2

== system IEEE14_case/AC_1/d_iq_line_13_14_block ==
  note: d_iq_line_13_14 in case14gfl
      | $1083.24555609096\,\mathrm{vq}_{\mathrm{bus},13}-185.159162902627\,\mathrm{iq}_{\mathrm{line},13,14}-376.991118430775\,\mathrm{id}_{\mathrm{line},13,14}-1083.24555609096\,\mathrm{vq}_{\mathrm{bus},14}$
      | Automatically generated on 2025-10-09 21:39:51 .
  State_id_line_13_14_fcef8 : Inport
  State_iq_line_13_14_4a60c : Inport  Port=2
  State_vq_bus_13_82621 : Inport  Port=3
  State_vq_bus_14_d664c : Inport  Port=4
  Add_331a6 : Sum
  Constant_-376.991118430775_7739d : Constant  Value=-376.991118430775
  Constant_1083.24555609096_a5034 : Constant  Value=1083.24555609096
  Constant_1083.24555609096_bdd8e : Constant  Value=1083.24555609096
  Constant_185.159162902627_5f783 : Constant  Value=185.159162902627
  Product_0f962 : Product
  Product_500bd : Product
  Product_95c35 : Product
  Product_b2662 : Product
  Subtract_0b3c0 : Sum  Inputs=+-
  Subtract_e80a9 : Sum  Inputs=+-
  Blockout_d_iq_line_13_14_49b1d : Outport
  wires:
  State_id_line_13_14_fcef8/1 -> Product_b2662/2
  Constant_-376.991118430775_7739d/1 -> Product_b2662/1
  Constant_185.159162902627_5f783/1 -> Product_95c35/1
  Product_95c35/1 -> Subtract_e80a9/2
  State_iq_line_13_14_4a60c/1 -> Product_95c35/2
  Product_b2662/1 -> Subtract_e80a9/1
  Constant_1083.24555609096_bdd8e/1 -> Product_0f962/1
  State_vq_bus_13_82621/1 -> Product_0f962/2
  Subtract_e80a9/1 -> Add_331a6/1
  Product_0f962/1 -> Add_331a6/2
  Product_500bd/1 -> Subtract_0b3c0/2
  Add_331a6/1 -> Subtract_0b3c0/1
  Constant_1083.24555609096_a5034/1 -> Product_500bd/1
  State_vq_bus_14_d664c/1 -> Product_500bd/2
  Subtract_0b3c0/1 -> Blockout_d_iq_line_13_14_49b1d/1

== system IEEE14_case/AC_1/d_iq_line_13_17_block ==
  note: d_iq_line_13_17 in case14gfl
      | $538.558740615393\,\mathrm{vq}_{\mathrm{bus},13}-32.3135244369236\,\mathrm{iq}_{\mathrm{line},13,17}-376.991118430775\,\mathrm{id}_{\mathrm{line},13,17}-538.558740615393\,\mathrm{vq}_{\mathrm{bus},17}$
      | Automatically generated on 2025-10-09 21:39:59 .
  State_id_line_13_17_62ede : Inport
  State_iq_line_13_17_7cac6 : Inport  Port=2
  State_vq_bus_13_d3788 : Inport  Port=3
  State_vq_bus_17_e9502 : Inport  Port=4
  Add_15de8 : Sum
  Constant_-376.991118430775_65d98 : Constant  Value=-376.991118430775
  Constant_32.3135244369236_02c63 : Constant  Value=32.3135244369236
  Constant_538.558740615393_91578 : Constant  Value=538.558740615393
  Constant_538.558740615393_9a531 : Constant  Value=538.558740615393
  Product_01512 : Product
  Product_2810d : Product
  Product_5b73c : Product
  Product_fd995 : Product
  Subtract_b8f55 : Sum  Inputs=+-
  Subtract_bda59 : Sum  Inputs=+-
  Blockout_d_iq_line_13_17_2fa46 : Outport
  wires:
  State_id_line_13_17_62ede/1 -> Product_5b73c/2
  Constant_-376.991118430775_65d98/1 -> Product_5b73c/1
  Constant_32.3135244369236_02c63/1 -> Product_2810d/1
  Product_fd995/1 -> Add_15de8/2
  Constant_538.558740615393_9a531/1 -> Product_fd995/1
  State_iq_line_13_17_7cac6/1 -> Product_2810d/2
  Product_2810d/1 -> Subtract_bda59/2
  Product_5b73c/1 -> Subtract_bda59/1
  State_vq_bus_13_d3788/1 -> Product_fd995/2
  Subtract_bda59/1 -> Add_15de8/1
  Product_01512/1 -> Subtract_b8f55/2
  Constant_538.558740615393_91578/1 -> Product_01512/1
  State_vq_bus_17_e9502/1 -> Product_01512/2
  Add_15de8/1 -> Subtract_b8f55/1
  Subtract_b8f55/1 -> Blockout_d_iq_line_13_17_2fa46/1

== system IEEE14_case/AC_1/d_iq_line_14_18_block ==
  note: d_iq_line_14_18 in case14gfl
      | $538.558740615393\,\mathrm{vq}_{\mathrm{bus},14}-32.3135244369236\,\mathrm{iq}_{\mathrm{line},14,18}-376.991118430775\,\mathrm{id}_{\mathrm{line},14,18}-538.558740615393\,\mathrm{vq}_{\mathrm{bus},18}$
      | Automatically generated on 2025-10-09 21:40:01 .
  State_id_line_14_18_708e0 : Inport
  State_iq_line_14_18_dd432 : Inport  Port=2
  State_vq_bus_14_bc785 : Inport  Port=3
  State_vq_bus_18_e3293 : Inport  Port=4
  Add_4f7ec : Sum
  Constant_-376.991118430775_1d6b4 : Constant  Value=-376.991118430775
  Constant_32.3135244369236_1ec0b : Constant  Value=32.3135244369236
  Constant_538.558740615393_8ba3c : Constant  Value=538.558740615393
  Constant_538.558740615393_f1fb8 : Constant  Value=538.558740615393
  Product_34246 : Product
  Product_37a8e : Product
  Product_4e9b4 : Product
  Product_ee7f0 : Product
  Subtract_2a28d : Sum  Inputs=+-
  Subtract_2a480 : Sum  Inputs=+-
  Blockout_d_iq_line_14_18_2b84d : Outport
  wires:
  Constant_-376.991118430775_1d6b4/1 -> Product_37a8e/1
  Constant_32.3135244369236_1ec0b/1 -> Product_34246/1
  Product_34246/1 -> Subtract_2a28d/2
  State_id_line_14_18_708e0/1 -> Product_37a8e/2
  State_iq_line_14_18_dd432/1 -> Product_34246/2
  Product_37a8e/1 -> Subtract_2a28d/1
  Constant_538.558740615393_8ba3c/1 -> Product_4e9b4/1
  State_vq_bus_14_bc785/1 -> Product_4e9b4/2
  Subtract_2a28d/1 -> Add_4f7ec/1
  Product_4e9b4/1 -> Add_4f7ec/2
  Product_ee7f0/1 -> Subtract_2a480/2
  Constant_538.558740615393_f1fb8/1 -> Product_ee7f0/1
  State_vq_bus_18_e3293/1 -> Product_ee7f0/2
  Add_4f7ec/1 -> Subtract_2a480/1
  Subtract_2a480/1 -> Blockout_d_iq_line_14_18_2b84d/1

== system IEEE14_case/AC_1/d_iq_line_1_2_block ==
  note: d_iq_line_1_2 in case14gfl
      | $6371.32192717213\,\mathrm{vq}_{\mathrm{bus},1}-123.476218948596\,\mathrm{iq}_{\mathrm{line},1,2}-376.991118430775\,\mathrm{id}_{\mathrm{line},1,2}-6371.32192717213\,\mathrm{vq}_{\mathrm{bus},2}$
      | Automatically generated on 2025-10-09 21:39:12 .
  State_id_line_1_2_008aa : Inport
  State_iq_line_1_2_a6f16 : Inport  Port=2
  State_vq_bus_1_f6968 : Inport  Port=3
  State_vq_bus_2_0b7a1 : Inport  Port=4
  Add_279ec : Sum
  Constant_-376.991118430775_62f78 : Constant  Value=-376.991118430775
  Constant_123.476218948596_36195 : Constant  Value=123.476218948596
  Constant_6371.32192717213_02e74 : Constant  Value=6371.32192717213
  Constant_6371.32192717213_bf3ee : Constant  Value=6371.32192717213
  Product_09986 : Product
  Product_4a37d : Product
  Product_7c274 : Product
  Product_cb76f : Product
  Subtract_21c93 : Sum  Inputs=+-
  Subtract_31c3e : Sum  Inputs=+-
  Blockout_d_iq_line_1_2_8e65d : Outport
  wires:
  Constant_-376.991118430775_62f78/1 -> Product_7c274/1
  Product_7c274/1 -> Subtract_31c3e/1
  State_id_line_1_2_008aa/1 -> Product_7c274/2
  Constant_123.476218948596_36195/1 -> Product_cb76f/1
  Product_cb76f/1 -> Subtract_31c3e/2
  State_iq_line_1_2_a6f16/1 -> Product_cb76f/2
  Product_09986/1 -> Add_279ec/2
  Constant_6371.32192717213_02e74/1 -> Product_09986/1
  State_vq_bus_1_f6968/1 -> Product_09986/2
  Subtract_31c3e/1 -> Add_279ec/1
  Constant_6371.32192717213_bf3ee/1 -> Product_4a37d/1
  State_vq_bus_2_0b7a1/1 -> Product_4a37d/2
  Add_279ec/1 -> Subtract_21c93/1
  Product_4a37d/1 -> Subtract_21c93/2
  Subtract_21c93/1 -> Blockout_d_iq_line_1_2_8e65d/1

== system IEEE14_case/AC_1/d_iq_line_1_5_block ==
  note: d_iq_line_1_5 in case14gfl
      | $1690.23994992277\,\mathrm{vq}_{\mathrm{bus},1}-91.3236644943274\,\mathrm{iq}_{\mathrm{line},1,5}-376.991118430775\,\mathrm{id}_{\mathrm{line},1,5}-1690.23994992277\,\mathrm{vq}_{\mathrm{bus},5}$
      | Automatically generated on 2025-10-09 21:39:14 .
  State_id_line_1_5_6753b : Inport
  State_iq_line_1_5_cd4fe : Inport  Port=2
  State_vq_bus_1_1731e : Inport  Port=3
  State_vq_bus_5_25d28 : Inport  Port=4
  Add_a7b19 : Sum
  Constant_-376.991118430775_79f91 : Constant  Value=-376.991118430775
  Constant_1690.23994992277_99aee : Constant  Value=1690.23994992277
  Constant_1690.23994992277_f0dc2 : Constant  Value=1690.23994992277
  Constant_91.3236644943274_00d61 : Constant  Value=91.3236644943274
  Product_0a1be : Product
  Product_420b7 : Product
  Product_8046a : Product
  Product_cbadd : Product
  Subtract_28c33 : Sum  Inputs=+-
  Subtract_9c3ad : Sum  Inputs=+-
  Blockout_d_iq_line_1_5_d4afd : Outport
  wires:
  Subtract_9c3ad/1 -> Add_a7b19/1
  Constant_-376.991118430775_79f91/1 -> Product_cbadd/1
  State_id_line_1_5_6753b/1 -> Product_cbadd/2
  Constant_91.3236644943274_00d61/1 -> Product_8046a/1
  Product_420b7/1 -> Add_a7b19/2
  Constant_1690.23994992277_99aee/1 -> Product_420b7/1
  State_iq_line_1_5_cd4fe/1 -> Product_8046a/2
  Product_cbadd/1 -> Subtract_9c3ad/1
  State_vq_bus_1_1731e/1 -> Product_420b7/2
  Product_8046a/1 -> Subtract_9c3ad/2
  Product_0a1be/1 -> Subtract_28c33/2
  Constant_1690.23994992277_f0dc2/1 -> Product_0a1be/1
  State_vq_bus_5_25d28/1 -> Product_0a1be/2
  Add_a7b19/1 -> Subtract_28c33/1
  Subtract_28c33/1 -> Blockout_d_iq_line_1_5_d4afd/1

== system IEEE14_case/AC_1/d_iq_line_2_3_block ==
  note: d_iq_line_2_3 in case14gfl
      | $1904.28407552041\,\mathrm{vq}_{\mathrm{bus},2}-89.482308708704\,\mathrm{iq}_{\mathrm{line},2,3}-376.991118430775\,\mathrm{id}_{\mathrm{line},2,3}-1904.28407552041\,\mathrm{vq}_{\mathrm{bus},3}$
      | Automatically generated on 2025-10-09 21:39:16 .
  State_id_line_2_3_74cbb : Inport
  State_iq_line_2_3_6a30b : Inport  Port=2
  State_vq_bus_2_4a159 : Inport  Port=3
  State_vq_bus_3_fc550 : Inport  Port=4
  Add_ca720 : Sum
  Constant_-376.991118430775_06b5f : Constant  Value=-376.991118430775
  Constant_1904.28407552041_35ca5 : Constant  Value=1904.28407552041
  Constant_1904.28407552041_43113 : Constant  Value=1904.28407552041
  Constant_89.482308708704_18ef1 : Constant  Value=89.482308708704
  Product_0812f : Product
  Product_281be : Product
  Product_87e25 : Product
  Product_e32fc : Product
  Subtract_437e9 : Sum  Inputs=+-
  Subtract_fea77 : Sum  Inputs=+-
  Blockout_d_iq_line_2_3_79888 : Outport
  wires:
  Constant_-376.991118430775_06b5f/1 -> Product_e32fc/1
  Constant_89.482308708704_18ef1/1 -> Product_87e25/1
  Product_87e25/1 -> Subtract_437e9/2
  State_id_line_2_3_74cbb/1 -> Product_e32fc/2
  State_iq_line_2_3_6a30b/1 -> Product_87e25/2
  Product_e32fc/1 -> Subtract_437e9/1
  Constant_1904.28407552041_35ca5/1 -> Product_0812f/1
  State_vq_bus_2_4a159/1 -> Product_0812f/2
  Subtract_437e9/1 -> Add_ca720/1
  Product_0812f/1 -> Add_ca720/2
  Product_281be/1 -> Subtract_fea77/2
  Constant_1904.28407552041_43113/1 -> Product_281be/1
  State_vq_bus_3_fc550/1 -> Product_281be/2
  Add_ca720/1 -> Subtract_fea77/1
  Subtract_fea77/1 -> Blockout_d_iq_line_2_3_79888/1

== system IEEE14_case/AC_1/d_iq_line_2_4_block ==
  note: d_iq_line_2_4 in case14gfl
      | $2138.10752286057\,\mathrm{vq}_{\mathrm{bus},2}-124.245428153428\,\mathrm{iq}_{\mathrm{line},2,4}-376.991118430775\,\mathrm{id}_{\mathrm{line},2,4}-2138.10752286057\,\mathrm{vq}_{\mathrm{bus},4}$
      | Automatically generated on 2025-10-09 21:39:18 .
  State_id_line_2_4_5b6e3 : Inport
  State_iq_line_2_4_af312 : Inport  Port=2
  State_vq_bus_2_24316 : Inport  Port=3
  State_vq_bus_4_4a861 : Inport  Port=4
  Add_b25a5 : Sum
  Constant_-376.991118430775_d327f : Constant  Value=-376.991118430775
  Constant_124.245428153428_a1294 : Constant  Value=124.245428153428
  Constant_2138.10752286057_75ac7 : Constant  Value=2138.10752286057
  Constant_2138.10752286057_af150 : Constant  Value=2138.10752286057
  Product_893d2 : Product
  Product_9ed8a : Product
  Product_b160d : Product
  Product_da8c9 : Product
  Subtract_0a8b3 : Sum  Inputs=+-
  Subtract_54b19 : Sum  Inputs=+-
  Blockout_d_iq_line_2_4_8ffa8 : Outport
  wires:
  Subtract_54b19/1 -> Blockout_d_iq_line_2_4_8ffa8/1
  State_vq_bus_2_24316/1 -> Product_893d2/2
  Constant_-376.991118430775_d327f/1 -> Product_9ed8a/1
  Product_893d2/1 -> Add_b25a5/2
  Constant_2138.10752286057_af150/1 -> Product_893d2/1
  State_id_line_2_4_5b6e3/1 -> Product_9ed8a/2
  Constant_124.245428153428_a1294/1 -> Product_b160d/1
  Product_b160d/1 -> Subtract_0a8b3/2
  State_iq_line_2_4_af312/1 -> Product_b160d/2
  Product_9ed8a/1 -> Subtract_0a8b3/1
  Subtract_0a8b3/1 -> Add_b25a5/1
  Product_da8c9/1 -> Subtract_54b19/2
  Constant_2138.10752286057_75ac7/1 -> Product_da8c9/1
  State_vq_bus_4_4a861/1 -> Product_da8c9/2
  Add_b25a5/1 -> Subtract_54b19/1

== system IEEE14_case/AC_1/d_iq_line_2_5_block ==
  note: d_iq_line_2_5 in case14gfl
      | $2168.11087204265\,\mathrm{vq}_{\mathrm{bus},2}-123.473914162829\,\mathrm{iq}_{\mathrm{line},2,5}-376.991118430775\,\mathrm{id}_{\mathrm{line},2,5}-2168.11087204265\,\mathrm{vq}_{\mathrm{bus},5}$
      | Automatically generated on 2025-10-09 21:39:20 .
  State_id_line_2_5_ba290 : Inport
  State_iq_line_2_5_dd836 : Inport  Port=2
  State_vq_bus_2_080ca : Inport  Port=3
  State_vq_bus_5_3bd85 : Inport  Port=4
  Add_d6cc2 : Sum
  Constant_-376.991118430775_35b94 : Constant  Value=-376.991118430775
  Constant_123.473914162829_636a5 : Constant  Value=123.473914162829
  Constant_2168.11087204265_1008a : Constant  Value=2168.11087204265
  Constant_2168.11087204265_485f1 : Constant  Value=2168.11087204265
  Product_10261 : Product
  Product_4448b : Product
  Product_686ea : Product
  Product_bb840 : Product
  Subtract_ece65 : Sum  Inputs=+-
  Subtract_ed576 : Sum  Inputs=+-
  Blockout_d_iq_line_2_5_1f062 : Outport
  wires:
  Constant_-376.991118430775_35b94/1 -> Product_686ea/1
  Constant_123.473914162829_636a5/1 -> Product_10261/1
  Product_10261/1 -> Subtract_ed576/2
  Product_686ea/1 -> Subtract_ed576/1
  State_id_line_2_5_ba290/1 -> Product_686ea/2
  State_iq_line_2_5_dd836/1 -> Product_10261/2
  Product_bb840/1 -> Add_d6cc2/2
  Constant_2168.11087204265_485f1/1 -> Product_bb840/1
  State_vq_bus_2_080ca/1 -> Product_bb840/2
  Subtract_ed576/1 -> Add_d6cc2/1
  Constant_2168.11087204265_1008a/1 -> Product_4448b/1
  State_vq_bus_5_3bd85/1 -> Product_4448b/2
  Add_d6cc2/1 -> Subtract_ece65/1
  Product_4448b/1 -> Subtract_ece65/2
  Subtract_ece65/1 -> Blockout_d_iq_line_2_5_1f062/1

== system IEEE14_case/AC_1/d_iq_line_3_4_block ==
  note: d_iq_line_3_4 in case14gfl
      | $2204.23971484988\,\mathrm{vq}_{\mathrm{bus},3}-147.706103292091\,\mathrm{iq}_{\mathrm{line},3,4}-376.991118430775\,\mathrm{id}_{\mathrm{line},3,4}-2204.23971484988\,\mathrm{vq}_{\mathrm{bus},4}$
      | Automatically generated on 2025-10-09 21:39:22 .
  State_id_line_3_4_7c07a : Inport
  State_iq_line_3_4_fc92d : Inport  Port=2
  State_vq_bus_3_c19a2 : Inport  Port=3
  State_vq_bus_4_4eaa9 : Inport  Port=4
  Add_3feaf : Sum
  Constant_-376.991118430775_0b544 : Constant  Value=-376.991118430775
  Constant_147.706103292091_07a39 : Constant  Value=147.706103292091
  Constant_2204.23971484988_0f7f6 : Constant  Value=2204.23971484988
  Constant_2204.23971484988_b64e4 : Constant  Value=2204.23971484988
  Product_53aba : Product
  Product_5debf : Product
  Product_e51ed : Product
  Product_f89ab : Product
  Subtract_2ee19 : Sum  Inputs=+-
  Subtract_e7d6e : Sum  Inputs=+-
  Blockout_d_iq_line_3_4_fcd14 : Outport
  wires:
  Constant_-376.991118430775_0b544/1 -> Product_e51ed/1
  State_id_line_3_4_7c07a/1 -> Product_e51ed/2
  Constant_147.706103292091_07a39/1 -> Product_5debf/1
  State_iq_line_3_4_fc92d/1 -> Product_5debf/2
  Product_e51ed/1 -> Subtract_2ee19/1
  Product_5debf/1 -> Subtract_2ee19/2
  State_vq_bus_3_c19a2/1 -> Product_53aba/2
  Product_53aba/1 -> Add_3feaf/2
  Constant_2204.23971484988_0f7f6/1 -> Product_53aba/1
  Subtract_2ee19/1 -> Add_3feaf/1
  Product_f89ab/1 -> Subtract_e7d6e/2
  Constant_2204.23971484988_b64e4/1 -> Product_f89ab/1
  State_vq_bus_4_4eaa9/1 -> Product_f89ab/2
  Add_3feaf/1 -> Subtract_e7d6e/1
  Subtract_e7d6e/1 -> Blockout_d_iq_line_3_4_fcd14/1

== system IEEE14_case/AC_1/d_iq_line_4_5_block ==
  note: d_iq_line_4_5 in case14gfl
      | $8952.53190289183\,\mathrm{vq}_{\mathrm{bus},4}-119.516300903606\,\mathrm{iq}_{\mathrm{line},4,5}-376.991118430775\,\mathrm{id}_{\mathrm{line},4,5}-8952.53190289183\,\mathrm{vq}_{\mathrm{bus},5}$
      | Automatically generated on 2025-10-09 21:39:24 .
  State_id_line_4_5_b6bf8 : Inport
  State_iq_line_4_5_0332d : Inport  Port=2
  State_vq_bus_4_22b10 : Inport  Port=3
  State_vq_bus_5_79571 : Inport  Port=4
  Add_e37d5 : Sum
  Constant_-376.991118430775_768e5 : Constant  Value=-376.991118430775
  Constant_119.516300903606_91f2c : Constant  Value=119.516300903606
  Constant_8952.53190289183_27c41 : Constant  Value=8952.53190289183
  Constant_8952.53190289183_ab934 : Constant  Value=8952.53190289183
  Product_0b9b7 : Product
  Product_26785 : Product
  Product_2f91f : Product
  Product_97980 : Product
  Subtract_3e6d1 : Sum  Inputs=+-
  Subtract_f99f3 : Sum  Inputs=+-
  Blockout_d_iq_line_4_5_de0fa : Outport
  wires:
  Constant_-376.991118430775_768e5/1 -> Product_2f91f/1
  Constant_8952.53190289183_27c41/1 -> Product_26785/1
  Subtract_f99f3/1 -> Blockout_d_iq_line_4_5_de0fa/1
  State_id_line_4_5_b6bf8/1 -> Product_2f91f/2
  Constant_119.516300903606_91f2c/1 -> Product_0b9b7/1
  Product_0b9b7/1 -> Subtract_3e6d1/2
  State_iq_line_4_5_0332d/1 -> Product_0b9b7/2
  Product_2f91f/1 -> Subtract_3e6d1/1
  State_vq_bus_4_22b10/1 -> Product_26785/2
  Subtract_3e6d1/1 -> Add_e37d5/1
  Product_26785/1 -> Add_e37d5/2
  Product_97980/1 -> Subtract_f99f3/2
  Constant_8952.53190289183_ab934/1 -> Product_97980/1
  State_vq_bus_5_79571/1 -> Product_97980/2
  Add_e37d5/1 -> Subtract_f99f3/1

== system IEEE14_case/AC_1/d_iq_line_4_7_block ==
  note: d_iq_line_4_7 in case14gfl
      | $1843.30284639447\,\mathrm{vq}_{\mathrm{bus},4}-376.991118430775\,\mathrm{id}_{\mathrm{line},4,7}-1843.30284639447\,\mathrm{vq}_{\mathrm{bus},7}$
      | Automatically generated on 2025-10-09 21:39:26 .
  State_id_line_4_7_b85c3 : Inport
  State_vq_bus_4_757cb : Inport  Port=2
  State_vq_bus_7_17236 : Inport  Port=3
  Add_aee87 : Sum
  Constant_-376.991118430775_43f4c : Constant  Value=-376.991118430775
  Constant_1843.30284639447_02a27 : Constant  Value=1843.30284639447
  Constant_1843.30284639447_22106 : Constant  Value=1843.30284639447
  Product_1161c : Product
  Product_14ee0 : Product
  Product_71122 : Product
  Subtract_719fc : Sum  Inputs=+-
  Blockout_d_iq_line_4_7_8270d : Outport
  wires:
  Constant_-376.991118430775_43f4c/1 -> Product_14ee0/1
  Product_1161c/1 -> Subtract_719fc/2
  Constant_1843.30284639447_02a27/1 -> Product_1161c/1
  Product_14ee0/1 -> Add_aee87/1
  State_id_line_4_7_b85c3/1 -> Product_14ee0/2
  Constant_1843.30284639447_22106/1 -> Product_71122/1
  Product_71122/1 -> Add_aee87/2
  State_vq_bus_4_757cb/1 -> Product_71122/2
  State_vq_bus_7_17236/1 -> Product_1161c/2
  Add_aee87/1 -> Subtract_719fc/1
  Subtract_719fc/1 -> Blockout_d_iq_line_4_7_8270d/1
